simulink model "ModeloMuelle"  (R2023b)
settings: Solver=VariableStepAuto  StartTime=0  StopTime=50  RelTol=1e-3
values from neighbouring files (symbols this model uses):
  dx0 = 0    [EjerciciosModelosContinuos.m]
  k = 0.5    [EjerciciosModelosContinuos.m]
  m = 5    [EjerciciosModelosContinuos.m]
  x0 = 0    [EjerciciosModelosContinuos.m]
settings Model: Creator=alfre  LastModifiedBy=alfre

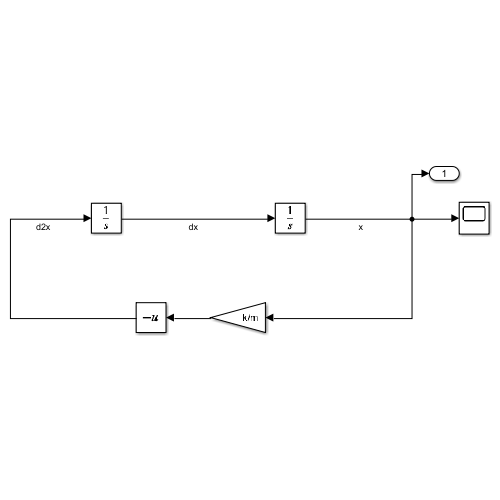
[thumbnail: Simulink's stored preview of the top-level diagram]
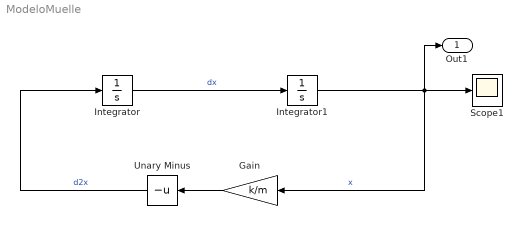
== system ModeloMuelle ==
  Gain : Gain  Gain=k/m
  Integrator : Integrator  InitialCondition=dx0
  Integrator1 : Integrator  InitialCondition=x0
  Scope1 : Scope
  Unary Minus : UnaryMinus
  Out1 : Outport
  wires:
  Integrator/1 -> Integrator1/1  "dx"
  Integrator1/1 -> Out1/1, Gain/1, Scope1/1  "x"
  Gain/1 -> Unary Minus/1
  Unary Minus/1 -> Integrator/1  "d2x"
